simulink model "QCar"  (R2025a)
settings: Solver=ode23t  StartTime=0.0  StopTime=8  MaxStep=0.005  RelTol=1e-3  AbsTol=1e-6
values from neighbouring files (symbols this model uses):
  cs = 1400    [build_quarter_car.m]
  Kd = 800    [build_quarter_car.m]
  Kp = 2000    [build_quarter_car.m]
undefined symbols (not defined in the file or in its folder): F_bump
libraries: fl_lib x10, nesl_utility x5
settings Model: Creator=soorajkrishnan  LastModifiedBy=soorajkrishnan

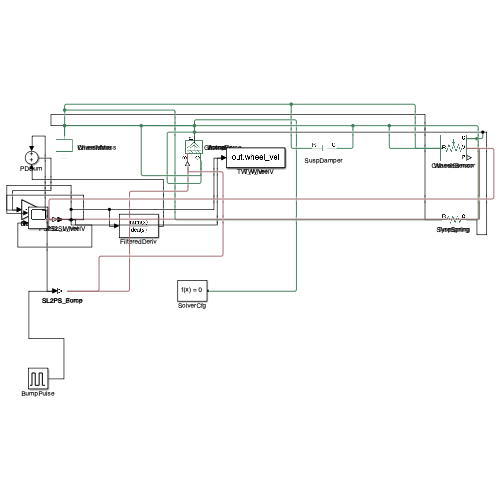
[thumbnail: Simulink's stored preview of the top-level diagram]
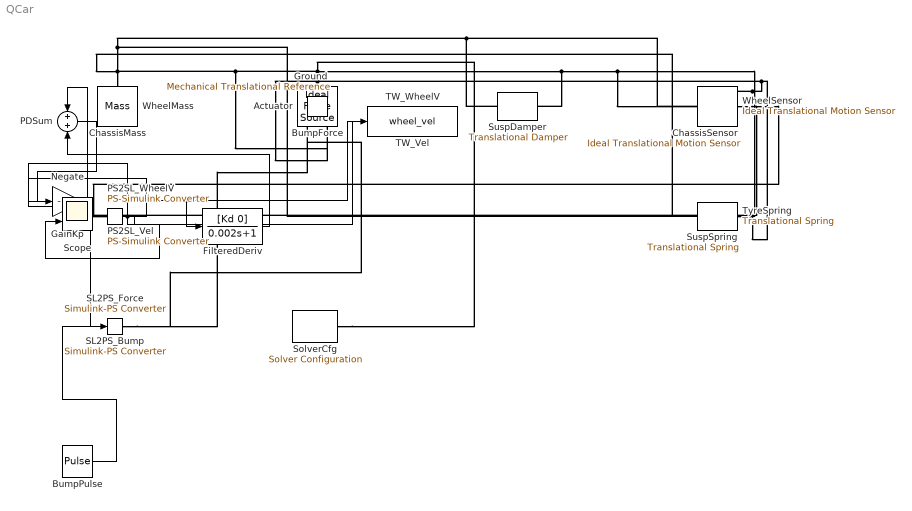
== system QCar ==
  Actuator : fl_lib/Mechanical/Mechanical Sources/Ideal Force Source
  BumpForce : fl_lib/Mechanical/Mechanical Sources/Ideal Force Source
  BumpPulse : DiscretePulseGenerator  PulseType=Time based  Amplitude=F_bump  Period=10  PulseWidth=0.5  PhaseDelay=0.5
  ChassisMass : fl_lib/Mechanical/Translational Elements/Mass  mass=ms kg  num_ports=foundation.enum.numPorts2.one  v_specify=off  v_priority=High  v=0 m/s  v_nominal_specify=off  v_nominal_value=1  v_nominal_unit=m/s  f_specify=off  f_priority=None  f=0 N  f_nominal_specify=off  f_nominal_value=1  f_nominal_unit=N
  ChassisSensor : fl_lib/Mechanical/Mechanical Sensors/Ideal Translational Motion Sensor  reference=foundation.enum.MeasurementReference.difference  acceleration_port=false  velocity_port=true  position_port=true  offset=0 m
  FilteredDeriv : TransferFcn  Numerator=[Kd 0]  Denominator=[0.002 1]
  GainKp : Gain  Gain=Kp
  Ground : fl_lib/Mechanical/Translational Elements/Mechanical Translational Reference
  Negate : Gain  Gain=-1
  PDSum : Sum
  PS2SL_Vel : nesl_utility/PS-Simulink Converter  PhysicalDomain=network_engine_domain  SubClassName=ps_output  LeftPortType=input  RightPortType=output  PseudoPeriodic=off  Frequencies=[]  VectorFormat=inherit  Unit=inherit  AffineConversion=off
  PS2SL_WheelV : nesl_utility/PS-Simulink Converter  PhysicalDomain=network_engine_domain  SubClassName=ps_output  LeftPortType=input  RightPortType=output  PseudoPeriodic=off  Frequencies=[]  VectorFormat=inherit  Unit=inherit  AffineConversion=off
  SL2PS_Bump : nesl_utility/Simulink-PS Converter  PhysicalDomain=network_engine_domain  SubClassName=ps_input  LeftPortType=input  RightPortType=output  PseudoPeriodic=off  Frequencies=[]  NoiseDistribution=none  NoiseParameters=[]  Unit=1  AffineConversion=off  FilteringAndDerivatives=provide  SimscapeFilterOrder=1  InputFilterTimeConstant=0.001  UdotUserProvided=0
  SL2PS_Force : nesl_utility/Simulink-PS Converter  PhysicalDomain=network_engine_domain  SubClassName=ps_input  LeftPortType=input  RightPortType=output  PseudoPeriodic=off  Frequencies=[]  NoiseDistribution=none  NoiseParameters=[]  Unit=1  AffineConversion=off  FilteringAndDerivatives=provide  SimscapeFilterOrder=1  InputFilterTimeConstant=0.001  UdotUserProvided=0
  Scope : Scope  NumInputPorts=2
  SolverCfg : nesl_utility/Solver Configuration  PhysicalDomain=network_engine_domain  SubClassName=solver  LeftPortType=input  RightPortType=generic  Tones=[]  Harmonics=[]  SimulateNoise=off  Profile=off  UseLocalSampling=off  EnableSwitchedLinearOptims=on  FrequencyDomain=off  UseCCode=off  RelTol=0.001  AbsTol=0.001  MinStep=1e-09  ToWorkspace=off  RevertToSquareIcSolve=off  NumHomotopyIterations=100  PhasorMode=off  PhasorModeNumHarmonics=1  ConsistencySolver=NEWTON_XTOL_AFTER_FTOL  IndexReductionMethod=DerivativeReplacement  DoDC=off  ResidualTolerance=1e-09  ConsistencyTolSource=GLOBAL  ConsistencyAbsTol=0.001  ConsistencyRelTol=0.001  ConsistencyTolFactor=0.001  UseLocalSolver=off  LocalSolverChoice=NE_BACKWARD_EULER_ADVANCER  ResolveIndetEquations=on  FunctionEvalNumThread=1  LocalSolverSampleTime=0.001  DoFixedCost=off  MaxNonlinIter=3  MaxModeIter=2  ComputeImpulses=off  ImpulseIterations=2  LinearAlgebra=auto  LinearAlgebraNumThread=0  EquationFormulation=NE_TIME_EF  DelaysMemoryBudget=1024  AutomaticFiltering=on  FilteringTimeConstant=0.001  PartitionStorageMethod=AS_NEEDED  PartitionMemoryBudget=1024  PartitionMethod=ROBUST  MultibodyUseLocalSolver=off  MultibodyLocalSolverChoice=ODE1  MultibodyLocalSolverSampleTime=0.001
  SuspDamper : fl_lib/Mechanical/Translational Elements/Translational Damper  D=cs N*s/m  v_specify=off  v_priority=None  v=0 m/s  v_nominal_specify=off  v_nominal_value=1  v_nominal_unit=m/s  f_specify=off  f_priority=None  f=0 N  f_nominal_specify=off  f_nominal_value=1  f_nominal_unit=N
  SuspSpring : fl_lib/Mechanical/Translational Elements/Translational Spring  spr_rate=ks N/m  v_specify=off  v_priority=None  v=0 m/s  v_nominal_specify=off  v_nominal_value=1  v_nominal_unit=m/s  f_specify=off  f_priority=None  f=0 N  f_nominal_specify=off  f_nominal_value=1  f_nominal_unit=N  x_specify=off  x_priority=High  x=0 m  x_nominal_specify=off  x_nominal_value=1  x_nominal_unit=m
  TW_Vel : ToWorkspace  VariableName=chassis_vel  SampleTime=-1
  TW_WheelV : ToWorkspace  VariableName=wheel_vel  SampleTime=-1
  TyreSpring : fl_lib/Mechanical/Translational Elements/Translational Spring  spr_rate=kt N/m  v_specify=off  v_priority=None  v=0 m/s  v_nominal_specify=off  v_nominal_value=1  v_nominal_unit=m/s  f_specify=off  f_priority=None  f=0 N  f_nominal_specify=off  f_nominal_value=1  f_nominal_unit=N  x_specify=off  x_priority=High  x=0 m  x_nominal_specify=off  x_nominal_value=1  x_nominal_unit=m
  WheelMass : fl_lib/Mechanical/Translational Elements/Mass  mass=mu kg  num_ports=foundation.enum.numPorts2.one  v_specify=off  v_priority=High  v=0 m/s  v_nominal_specify=off  v_nominal_value=1  v_nominal_unit=m/s  f_specify=off  f_priority=None  f=0 N  f_nominal_specify=off  f_nominal_value=1  f_nominal_unit=N
  WheelSensor : fl_lib/Mechanical/Mechanical Sensors/Ideal Translational Motion Sensor  reference=foundation.enum.MeasurementReference.difference  acceleration_port=false  velocity_port=true  position_port=true  offset=0 m
  wires:
  BumpPulse/1 -> SL2PS_Bump/1
  PS2SL_Vel/1 -> FilteredDeriv/1, TW_Vel/1, Scope/1, GainKp/1
  GainKp/1 -> PDSum/1
  PDSum/1 -> Negate/1
  Negate/1 -> SL2PS_Force/1
  PS2SL_WheelV/1 -> TW_WheelV/1, Scope/2
  FilteredDeriv/1 -> PDSum/2
  connections:
  SolverCfg/RConn1 -- TyreSpring/RConn1 -- WheelSensor/RConn1 -- ChassisSensor/RConn1 -- Ground/LConn1 -- BumpForce/RConn2
  BumpForce/LConn1 -- WheelSensor/LConn1 -- SuspSpring/RConn1 -- SuspDamper/RConn1 -- Actuator/RConn2 -- WheelMass/LConn1 -- TyreSpring/LConn1
  SuspSpring/LConn1 -- ChassisSensor/LConn1 -- SuspDamper/LConn1 -- ChassisMass/LConn1 -- Actuator/LConn1
  ChassisSensor/RConn2 -- PS2SL_Vel/LConn1
  WheelSensor/RConn2 -- PS2SL_WheelV/LConn1
  SL2PS_Bump/RConn1 -- BumpForce/RConn1
  SL2PS_Force/RConn1 -- Actuator/RConn1
